simulink model "robotTask"  (R2012b)
settings: Solver=FixedStepDiscrete  StartTime=0.0  StopTime=10.0  FixedStep=0.001  RelTol=1e-3
undefined symbols (not defined in the file): acquireMethods, autoplayMovementDuration, autoplayReactionTime, autoplayRotationDuration, autoplayRotationStart, centerOffset, clickPercentage, clickRefractoryPeriod, clickTargetColor, clickTargetHoverColor, cuedText, cuedTextLength, cumulativeDwell, cursorColorClick, cursorColorClosed, cursorColorOpen, cursorDiameter, cursorNeuralColor, cursorNonneuralColor, delayOrder, delayPeriodGainScale, displayObject, doHeadSpeedFail, drawNumbersOnTargets, dwellRefractoryPeriod, errorAssistAxis, errorAssistR, errorAssistTheta, expRandBinSize, expRandMax, expRandMin, expRandMu, eyeMode, failOnLiftoff, failurePenalty, falseClickFails, fingerPositionTolerance, fixedSeqMode, freePlayMode, gain, gloveBias, gloveLPDenominator, gloveLPNumerator, gloveNonlinearCorrection, gloveXCorrection, gloveYCorrection, gridEdges, gridTilesEachDim, headSpeedCap, holdDuration, holdTime, initialInput, initialLockout, initialState, inputType, keyboard, keyboardDims, keyPressedTime, lockFingerPosition, maxTaskTime ... (+100)
(part 2 of 2)

== matlab function robotTask/robotTaskSplit ==
  data: xkRaw input double size=[double(xkConstants.NUM_STATE_DIMENSIONS) 1]; xkMod input; behaviorPacket input Bus: behaviorPacketBus size=1; vizData input Bus: peripheralData; clickState input; clickParameters input; taskOutput output Bus: taskOutput; stateParameters input Bus: stateParams size=1; taskParameters input Bus: taskParamsBus; clock input; xpcTET input; xkModBiasEst input; taskAgnosticXk input
function taskOutput  = robotTaskSplit(xkRaw, xkMod, behaviorPacket, vizData, clickState, clickParameters, stateParameters, taskParameters, clock, xpcTET, xkModBiasEst, taskAgnosticXk)
%#codegen
% This is the state-machine-like implementation of the robot task. 
% It was originally cloned from cursorTask, but my goal is to strip out the
% unused task logic in preparation for having future robotic tasks.
% 
% This also does some robot-specific things like using the click selection
% to implement grasp logic. 
%
% It two state inputs, xkRaw (which gets fed back to
% the decoder), and xkMod. Generally should look at xkMod for task logic,
% but if the game needs to change a state element which ought to propogate
% into the decoder (for example re-seed the cursor), it should do this to
% both xkRaw and xkMod.

% taskParameters is taskParamsBus, which is set by
% robotTask_buildWorkspace.m

robotPosition = behaviorPacket.robotPosition; % 1x3 of x y z % SDS I *think* but need to check that this is the returned position of robot
behaviorRequestClock = behaviorPacket.xpcRequestClock;
peripheralTimestamp = behaviorPacket.peripheralTimestamp(1:16);

%% CONSTANTS
TASK_NAME = 'robot';
VERSION_ID = single(1); % v1 is Feb 2017
NUM_DIMS = uint8(cursorConstants.NUM_DIMENSIONS); % dimensionality of the task. August 2016 raised this from 2 to 3
STATEVEC_SIZE = double( xkConstants.NUM_STATE_DIMENSIONS ); % SDS July 2016
INIT_LENGTH = uint16(100); %ms
PRE_TRIAL_LENGTH = uint16(20); %ms
INIT_TIME = uint32(2000);


%% INITIALIZE CURSOR TASK OUTPUT
fileLoggerData.data = uint8(zeros(1,1400));
fileLoggerData.dataLen = uint16(0);
fileLoggerData.fileName = uint8(zeros(1,20));
fileLoggerData.send = false;

fileLoggerFormat.format = uint8(zeros(1,1400));
fileLoggerFormat.formatLen = uint16(0);
fileLoggerFormat.fileName = uint8(zeros(1,20));

fileLoggerFormatAndData.format = fileLoggerFormat;
fileLoggerFormatAndData.data = fileLoggerData;

%% whether or not to allow the cursor to be stopped (e.g. during click)
allowStop = true;
resetHMM = false;

taskOutput.flushFiles = false;
taskOutput.sendFormat = false;
taskOutput.taskDetails = fileLoggerFormat;
taskOutput.discrete = fileLoggerFormatAndData;
taskOutput.continuous = fileLoggerFormatAndData;
taskOutput.screen = fileLoggerFormatAndData;
taskOutput.sound = fileLoggerFormatAndData;
taskOutput.asynch = fileLoggerFormatAndData;
taskOutput.ttl = double(0);
taskOutput.xk = xkRaw;
taskOutput.inputType = taskParameters.initialInput;
% initial target is off-screen
taskOutput.currentTarget = single(999.*ones([double(xkConstants.NUM_TARGET_DIMENSIONS) 1]));
taskOutput.state = uint16(CursorStates.STATE_INIT);
taskOutput.paused = false;
taskOutput.allowStop = allowStop;
taskOutput.resetHMM = resetHMM;

%% TASK DETAILS PACKET
taskOutput.taskDetails = packFileLoggerTaskDetails(TASK_NAME, VERSION_ID, ...
    'STATE_INIT', uint8(CursorStates.STATE_INIT), ...
    'STATE_PRE_TRIAL', uint8(CursorStates.STATE_PRE_TRIAL),...
    'STATE_NEW_TARGET', uint8(CursorStates.STATE_NEW_TARGET),...
    'STATE_MOVE', uint8(CursorStates.STATE_MOVE),...
    'STATE_ACQUIRE', uint8(CursorStates.STATE_ACQUIRE),...
    'STATE_SUCCESS', uint8(CursorStates.STATE_SUCCESS),...
    'STATE_FAIL', uint8(CursorStates.STATE_FAIL),...
    'STATE_CENTER_TARGET', uint8(CursorStates.STATE_CENTER_TARGET),...
    'STATE_END', uint8(CursorStates.STATE_END),...
    'STATE_RECENTER_DELAY', uint8(CursorStates.STATE_RECENTER_DELAY),...
    'STATE_MOVE_CLICK', uint8(CursorStates.STATE_MOVE_CLICK),...
    'STATE_MOVE_HOVER', uint8(CursorStates.STATE_HOVER),...
    'CLICK_IDLE', uint8(DiscreteStates.CLICK_IDLE),...
    'CLICK_MAIN', uint8(DiscreteStates.CLICK_MAIN),...
    'TARGET_TYPE_DWELL', uint8(cursorConstants.TARGET_TYPE_DWELL), ...
    'TARGET_TYPE_CLICK', uint8(cursorConstants.TARGET_TYPE_CLICK), ...
    'INPUT_TYPE_MOUSE_ABSOLUTE', uint8(cursorConstants.INPUT_TYPE_MOUSE_ABSOLUTE),...
    'INPUT_TYPE_DECODE_V', uint8(cursorConstants.INPUT_TYPE_DECODE_V),...
    'INPUT_TYPE_AUTO_PLAY', uint8(cursorConstants.INPUT_TYPE_AUTO_PLAY),...
    'CLICK_TYPE_NONE', uint8(clickConstants.CLICK_TYPE_NONE),...
    'CLICK_TYPE_NEURAL', uint8(clickConstants.CLICK_TYPE_NEURAL),...
    'OUTPUT_TYPE_CURSOR', uint8(cursorConstants.OUTPUT_TYPE_CURSOR),...
    'OUTPUT_TYPE_ROBOT', uint8(cursorConstants.OUTPUT_TYPE_ROBOT)...
);



%% DEFINE PERSISTENTS
persistent state vizPacket;
persistent pauseTriggered;
persistent stateTimer;
persistent holdTimer;
persistent clickTimer; %added SDS Jan 2017, so both click and hold can be used to do this task
persistent cursorColors;

persistent currentTarget;
persistent nextTarget;

persistent currentTargetType nextTargetType;  % dwell or click
persistent trialNum targetOrder cycleNum cycleIndex;
persistent trialDelayLength;

persistent localAcquired localTotal localTotalTime localAcqTime;
persistent acquireTime lastState;

persistent lockedParameters inputType outputType;
persistent stateBeforePreTrial;

persistent lastSoundTime;
persistent lastSoundState;

persistent initialCursorPosition previousInput;

persistent totalTaskTime;
persistent lastAcquireSuccess previousTarget;

%% INITIALIZE PERSISTENTS
if(isempty(state))
    state = uint16(CursorStates.STATE_INIT);
    lastState = state;
    % initial current target is off screen
    currentTarget = single(999.*ones([double(xkConstants.NUM_TARGET_DIMENSIONS) 1]));
    nextTarget = single(zeros([double(xkConstants.NUM_TARGET_DIMENSIONS) 1]));

    
    vizPacket = initVizPacket;
    stateTimer = uint16(0);
    holdTimer = int16(0);
    clickTimer = int16(0); % initialize
    pauseTriggered = true;
    
    cursorColors = double(zeros([3 2])); % there's a second cursor (column 2) allowed
    
    
    %% buffer all the parameters off the bus
    lockedParameters = taskParameters;
    
    
    inputType = lockedParameters.initialInput;
    
    targetOrder = uint16(zeros([1 double(cursorConstants.MAX_TARGETS)]));
    trialNum = uint16(0);
    cycleNum = uint16(0);
    cycleIndex = uint16(0);
    trialDelayLength = uint16(0);
    
    localTotal = uint16(0);
    localTotalTime = uint16(0);
    localAcquired = uint16(0);
    localAcqTime = uint16(0);
    localScore = uint16(0);
    totalScore = uint16(0);
    acquireTime = stateTimer;
    currentTargetType = uint16(cursorConstants.TARGET_TYPE_DWELL);
    nextTargetType = uint16(cursorConstants.TARGET_TYPE_DWELL);
	stateBeforePreTrial = uint16(0);
    lastSoundTime = clock;
    lastSoundState = uint8(CursorStates.SOUND_STATE_IDLE);
    
    initialCursorPosition = zeros(NUM_DIMS,1);
    previousInput = inputType;
    
    totalTaskTime = uint32(0);
    
    lastAcquireSuccess = false;
    previousTarget = currentTarget;
end


%% some initialization
if(clock < INIT_TIME)
    pauseTriggered = true;
end
outputType = lockedParameters.outputType; % determines what graphics engine will render this task.

% We usually shouldn't write discrete data
writeDiscreteData = false;
writeContinuousData = true;

if(vizData.receive && (vizData.dataLen > 0 ))
    vizPacket = parseVizPacket(vizData.data);
end

isNeural = (uint16(inputType) == uint16(cursorConstants.INPUT_TYPE_DECODE_V));
isClicked = (uint16(clickState) == uint16(DiscreteStates.CLICK_MAIN));
if ~isClicked
    clickTimer = int16(0); % resets t be not-clicked
end
isNone = (uint16(inputType) == uint16(cursorConstants.INPUT_TYPE_NONE));

% which state elements do I look to for the cursor's position? SDS July 2016
xk2HorizontalPos = uint8( lockedParameters.xk2HorizontalPos );
xk2VerticalPos = uint8( lockedParameters.xk2VerticalPos );
xk2HorizontalVel = uint8( lockedParameters.xk2HorizontalVel );
xk2VerticalVel = uint8( lockedParameters.xk2VerticalVel );
xk2DepthPos = uint8( lockedParameters.xk2DepthPos );
xk2DepthVel = uint8( lockedParameters.xk2DepthVel );
xk2RotatePos = uint8( lockedParameters.xk2RotatePos );
xk2RotateVel = uint8( lockedParameters.xk2RotateVel );
xk2Rotate2Pos = uint8( lockedParameters.xk2Rotate2Pos );
xk2Rotate2Vel = uint8( lockedParameters.xk2Rotate2Vel );

canBePosInds = [xk2HorizontalPos,xk2VerticalPos,xk2DepthPos,xk2RotatePos,xk2Rotate2Pos];
canBeVelInds = [xk2HorizontalVel,xk2VerticalVel,xk2DepthVel,xk2RotateVel,xk2Rotate2Vel];
effectorPosInds = canBePosInds(1:NUM_DIMS);
effectorVelInds = canBeVelInds(1:NUM_DIMS);

if uint16(outputType) == uint16(cursorConstants.OUTPUT_TYPE_ROBOT)
    effectorPos = double(robotPosition(1:2)); % MAKE N-D
    % TODO: when we start doing simulated/real arms, work on this stuff
elseif uint16(outputType) == uint16(cursorConstants.OUTPUT_TYPE_SCLCURSOR)
    effectorPos = xkMod(effectorPosInds);
else
    effectorPos = xkMod(effectorPosInds);
end


%% set the cursor color 
if isClicked
    cursorColors(1:end,1) = lockedParameters.cursorColorClick;%[255; 0; 0;];
elseif isNeural
    cursorColors(1:end,1) = [255; 255; 255;]; % white neural cursor
elseif isNone
    cursorColors(1:end,1) = [0; 204; 102;]; % is this used?
else
    cursorColors(1:end,1) = [255; 133; 0]; % orange autoplay cursor
end


targetColor = 'g';



if ~pauseTriggered
    totalTaskTime = totalTaskTime+1;
end

%% generally, allow cursor to stop off target. check options
allowStop = lockedParameters.stopOffTarget;

% STATE MACHINE
switch state
    %% STATE_INIT
    case {CursorStates.STATE_INIT}
        % set all the persistents that may have been changed by user input
        pauseTriggered = stateParameters.pause;
        lockedParameters = taskParameters;
        writeContinuousData = false;
        inputType = lockedParameters.initialInput;
        % generate some entropy
        jnk = rand(1,1);
        
        initialCursorPosition = xkMod(effectorPosInds(1:NUM_DIMS)); % handhold the compiler so it knows its fixed dim.
        if ~pauseTriggered
            stateTimer = stateTimer + 1;
        end
        if stateTimer >= INIT_LENGTH
            stateTimer = uint16(0);
            trialNum = uint16(0);
            % Initialize without a target, so jjust put it somewhere far
            % away            
            currentTarget(:) = int16(999.*ones(double(xkConstants.NUM_TARGET_DIMENSIONS),1));
            cycleNum = uint16(0);
            
            % For robot task, go straight to STATE_MOVE or
            % STATE_MOVE_CLICK
            %
            state = uint16( RobotStates.STATE_PRE_TRIAL );
            % Key logic for whether to go into STATE_MOVE or
            % STATE_MOVE_CLICK, based on what mode is selected,
%             if currentTargetType == cursorConstants.TARGET_TYPE_CLICK;
%                 state = uint16(RobotStates.STATE_MOVE_GRASP_OPEN);
%             elseif currentTargetType == cursorConstants.TARGET_TYPE_DWELL;
%                 state = uint16(RobotStates.STATE_MOVE);
%             end
        end
        
        
        %% STATE_CENTER_TARGET
    case {RobotStates.STATE_CENTER_TARGET}
        stateTimer = stateTimer + 1;
        initialCursorPosition = xkMod(effectorPosInds(1:NUM_DIMS)); % the (1:NUM_DIMS) is to handhold compilter about the dimensionality  
        if isCursorOnTarget(effectorPos, double(lockedParameters.cursorDiameter)/2, currentTarget, double(lockedParameters.targetDiameter)/2, NUM_DIMS)
            state = uint16(RobotStates.STATE_SUCCESS);
            stateTimer = uint16(0);
        end
        
        
        
        %% STATE_NEW_TARGET
    case {RobotStates.STATE_NEW_TARGET}
        holdTimer = int16(0); % reset hold timer. Needed now for Gridlike task logic SDS 15 Dec 2016
        
        if ~trialDelayLength
            if lockedParameters.useRandomDelay
                % pick a new random delay
                while double(trialDelayLength) < lockedParameters.expRandMin || double(trialDelayLength) > lockedParameters.expRandMax
                    trialDelayLength = uint16(lockedParameters.expRandMu * -log(rand([1 1])));
                end
                trialDelayLength = uint16(round(double(trialDelayLength) / double(lockedParameters.expRandBinSize))*lockedParameters.expRandBinSize);
            else
                trialDelayLength = uint16(lockedParameters.expRandMu);
            end
        end
        
        % Check whether cursor is in target differs for Gridlike task.
        cursorOnTarget = isCursorOnTarget(effectorPos, double(lockedParameters.cursorDiameter)/2,  currentTarget, double(lockedParameters.targetDiameter)/2, NUM_DIMS);
        
        stateTimer = stateTimer + 1;
        if stateTimer >= trialDelayLength
            % great, present the new target now
            stateTimer = uint16(0);
            previousTarget = currentTarget;
            currentTarget = nextTarget;
            currentTargetType = nextTargetType;

            % is recentering turned on, and does that apply here?
            if (lockedParameters.recenterOnSuccess && lastAcquireSuccess ==true ) || ...
                    (lockedParameters.recenterOnFail && lastAcquireSuccess == false)
                recenterThisTrial = true;
            else
                recenterThisTrial = false;
            end
            
            if recenterThisTrial
                state = uint16(RobotStates.STATE_RECENTER_DELAY);
            else
                if lockedParameters.soundOnGo
                    lastSoundTime = clock;
                    lastSoundState = uint8(RobotStates.SOUND_STATE_GO);
                end
                % Key logic for whether to go into STATE_MOVE or
                % one of the move-and-grasp states
                if currentTargetType == cursorConstants.TARGET_TYPE_CLICK;
                    state = uint16(RobotStates.STATE_MOVE_GRASP_OPEN);
                elseif currentTargetType == cursorConstants.TARGET_TYPE_DWELL;
                    state = uint16(RobotStates.STATE_MOVE);
                end
            end
        elseif ~cursorOnTarget 
            % Note that there's no stay-over-target rule for Gridlike
            % task, so in that task this won't be reached.
            % For other task variants: if cursor moves from last target too early,
            % just reset delay timer
            stateTimer = uint16(0);
        end
        
        %% STATE_RECENTER_DELAY
    case {RobotStates.STATE_RECENTER_DELAY}
        % (Gridlike task variant never enters this state)
        % Not currently used in robot task either.
        stateTimer = stateTimer + 1;
        if stateTimer <= lockedParameters.recenterDelay
            switch lockedParameters.taskType
                case {uint32(cursorConstants.TASK_PINBALL), ...
                        uint32(cursorConstants.TASK_CENTER_OUT)}                       
                    xkMod(effectorPosInds,1) = previousTarget(1:NUM_DIMS);
                    xkMod(effectorVelInds,1) = 0;
                case uint32(cursorConstants.TASK_CENTER_OUT_NO_BACK)
                    xkMod([effectorPosInds, effectorVelInds],1) = 0;
                case uint32(cursorConstants.TASK_NOTARGETS)
                    % go back to workspace center
                    xkMod([effectorPosInds, effectorVelInds],1) = 0;
            end
            xkRaw([effectorPosInds, effectorVelInds],1) = xkMod([effectorPosInds, effectorVelInds],1); % also lock xkRaw
        else
            if lockedParameters.soundOnGo
                lastSoundTime = clock;
                lastSoundState = uint8(RobotStates.SOUND_STATE_GO);
            end
            
            stateTimer = uint16(0);
            if currentTargetType == cursorConstants.TARGET_TYPE_CLICK;
                state = uint16(RobotStates.STATE_MOVE_GRASP_OPEN);
            elseif currentTargetType == cursorConstants.TARGET_TYPE_DWELL;
                state = uint16(RobotStates.STATE_MOVE);
            end
        end
        
        %% STATE_MOVE
    case {RobotStates.STATE_MOVE}
        % moving and no grasp control
        stateTimer = stateTimer + 1;
        inputType = lockedParameters.inputType; % needed to unlock cursor if not coming from success state
        

        cursorOnTarget = isCursorOnTarget(effectorPos, double(lockedParameters.cursorDiameter)/2,  currentTarget, double(lockedParameters.targetDiameter)/2, NUM_DIMS);

        if cursorOnTarget
            state = uint16(RobotStates.STATE_ACQUIRE);
            if holdTimer >= 0
                holdTimer = int16(0); % reset hold timer -- it could have been nonzero from either previous
                % target hold or time spent in any tile in Gridlike mode.
            else
                holdTimer = holdTimer; % allows negative to carry over for newTrialAddedDwell
            end
            
            if lockedParameters.soundOnOverTarget
                % if we're on autoplay, make a tapping noise
                lastSoundTime = clock;
                lastSoundState = uint8(RobotStates.SOUND_STATE_OVER_TARGET);
            end
        elseif stateTimer >= lockedParameters.trialTimeout
            stateTimer = uint16(0);
            state = uint16(RobotStates.STATE_FAIL);
        end

        
        
    %% STATE_MOVE_GRASP_OPEN
    case {RobotStates.STATE_MOVE_GRASP_OPEN}
        stateTimer = stateTimer + 1;
        inputType = lockedParameters.inputType; % needed to unlock if not coming from success
        
        
        networkOutput.discrete.send = false; % SDS: not really sure why this is set here but not in e.g. STATE_MOVE
        
        cursorOnTarget = isCursorOnTarget(effectorPos, double(lockedParameters.cursorDiameter)/2,  currentTarget, double(lockedParameters.targetDiameter)/2, NUM_DIMS);
        targetColor = 'y';
        % Shows hand should be open based on cursor color (useful for SCL
        % testing).
        cursorColors(1:end,1) = lockedParameters.cursorColorOpen;
        
        if clickState == uint16(DiscreteStates.CLICK_MAIN)
            clickTimer = clickTimer + 1;
            if clickTimer >= clickParameters.clickHoldTime && stateTimer > taskParameters.selectionRefractoryMS
                % Click command was sent into the task long enough that the
                % toggle is triggered, AND we've been in this state longer
                % than the refractory period (this debounces state
                % transitions).
                state = uint16( RobotStates.STATE_MOVE_GRASP_CLOSED );
                stateTimer = uint16(0);
            end
        end
        
        
        if cursorOnTarget
            state = uint16(RobotStates.STATE_HOVER);
            if holdTimer >= 0
                holdTimer = int16(0); % reset hold timer -- it could have been nonzero from either previous
                % target hold or time spent in any tile in Gridlike mode.
            else
                holdTimer = holdTimer; % allows negative to carry over for newTrialAddedDwell
            end
            
            if lockedParameters.soundOnOverTarget
                % if we're on autoplay, make a tapping noise
                lastSoundTime = clock;
                lastSoundState = uint8(RobotStates.SOUND_STATE_OVER_TARGET);
            end
            
        elseif stateTimer >= lockedParameters.trialTimeout
            stateTimer = uint16(0);
            state = uint16(RobotStates.STATE_FAIL);
        end
        
  %% STATE_MOVE_GRASP_CLOSED
    case {RobotStates.STATE_MOVE_GRASP_CLOSED}
        stateTimer = stateTimer + 1;
        inputType = lockedParameters.inputType; % needed to unlock if not coming from success
        
        
        networkOutput.discrete.send = false; % SDS: not really sure why this is set here but not in e.g. STATE_MOVE
        
        cursorOnTarget = isCursorOnTarget(effectorPos, double(lockedParameters.cursorDiameter)/2,  currentTarget, double(lockedParameters.targetDiameter)/2, NUM_DIMS);
        targetColor = 'y';
        % Shows hand should be open based on cursor color (useful for SCL
        % testing).
        cursorColors(1:end,1) = lockedParameters.cursorColorClosed;
        
         if clickState == uint16(DiscreteStates.CLICK_MAIN)
            clickTimer = clickTimer + 1;
            if clickTimer >= clickParameters.clickHoldTime && stateTimer > taskParameters.selectionRefractoryMS
                % Click command was sent into the task long enough that the
                % toggle is triggered, AND we've been in this state longer
                % than the refractory period (this debounces state
                % transitions).
                state = uint16( RobotStates.STATE_MOVE_GRASP_OPEN );
                stateTimer = uint16(0);
            end
        end
        
        if cursorOnTarget
            state = uint16(RobotStates.STATE_HOVER);
            if holdTimer >= 0
                holdTimer = int16(0); % reset hold timer -- it could have been nonzero from either previous
                % target hold or time spent in any tile in Gridlike mode.
            else
                holdTimer = holdTimer; % allows negative to carry over for newTrialAddedDwell
            end
            
            if lockedParameters.soundOnOverTarget
                % if we're on autoplay, make a tapping noise
                lastSoundTime = clock;
                lastSoundState = uint8(RobotStates.SOUND_STATE_OVER_TARGET);
            end
            
        elseif stateTimer >= lockedParameters.trialTimeout
            stateTimer = uint16(0);
            state = uint16(RobotStates.STATE_FAIL);
        end       
        
        %% STATE_HOVER
    case {RobotStates.STATE_HOVER}
        % Hover is being over a target when click enabled - Sergey
        stateTimer = stateTimer + 1;
        % SDS Jan 26 2017. I'm making hold to select possible in cursor
        % task, even when click is also an option. Hence, now holdTimer
        % counts up here too.
        holdTimer = holdTimer + 1;
        
        % if "stopOffTarget" is false, then we must manually
        %   flag times when cursor is over target to allow click to stop
        allowStop = true;
        
        networkOutput.discrete.send = false;
        
        cursorOnTarget = isCursorOnTarget(effectorPos, double(lockedParameters.cursorDiameter)/2,  currentTarget, double(lockedParameters.targetDiameter)/2, NUM_DIMS);
        targetColor = 'p';
        
        if clickState == uint16(DiscreteStates.CLICK_MAIN)
            clickTimer = clickTimer + 1;
            if clickTimer >= clickParameters.clickHoldTime % should be clickTimer
                if holdTimer > 0
                    % above check is the refractory period.
                    if cursorOnTarget
                        state = uint16(RobotStates.STATE_SUCCESS);
                        stateTimer = uint16(0);
                    else
                        state = uint16(RobotStates.STATE_FAIL);
                        stateTimer = uint16(0);
                        %  holdTimer = int16(0);  % should be clickTimer
                    end
                end
            end
            
        elseif ~cursorOnTarget
            % the elseif means that if mid-click and drifting off a
            % target, that's not yet a fail. But if NOT still clicking,
            % and drift off a target, then it goes to STATE_MOVE_CLICK.
            % Note that due to logic above in the click check, gridlike
            % task is less forgiving.
            state = uint16(RobotStates.STATE_MOVE_GRASP_OPEN);
            % TODO: need to think about what state to move to after an
            % incorrect grasp command. Maybe irrelevant if we don't end up
            % using this
            
            % we were over the target, but now we're not, so either
            % left target (vanilla cursor task) or the tile (gridlike).
            % Either way, hold timer becomes zero if nonnegative/
            if holdTimer > 0
                % this check > 0 is so that rapidly fluttering over
                % target in gridlike task doesn't nullify refractory
                % period.
                holdTimer = int16(0);
            end
        elseif holdTimer >= lockedParameters.holdTime
            % held over the target long enough to acquire it
            acquireTime = stateTimer;
            stateTimer = uint16(0);
            state = uint16(RobotStates.STATE_SUCCESS);
            holdTimer = int16(0);
            
        elseif stateTimer >= lockedParameters.trialTimeout
            stateTimer = uint16(0);
            state = uint16(RobotStates.STATE_FAIL);
            holdTimer = int16(0);  % should be clickTimer
            
        else
            clickTimer = int16(0);    % should be clickTimer
            % likely redundant to check at top of the function, but
            % can't hurt here.
        end
        
        %% STATE_ACQUIRE
    case {RobotStates.STATE_ACQUIRE}
        stateTimer = stateTimer + 1;
        holdTimer = holdTimer + 1;
        % if "stopOffTarget" is false, then we must manually
        %   flag times when cursor is over target to allow click to stop
        
        % Check whether cursor is in target differs for Gridlike task.
        cursorOnTarget = isCursorOnTarget(effectorPos, double(lockedParameters.cursorDiameter)/2,  currentTarget, double(lockedParameters.targetDiameter)/2, NUM_DIMS);
        targetColor = 'b';

        allowStop = true;
        
        if ~cursorOnTarget
            state = uint16(RobotStates.STATE_MOVE);
            if holdTimer > 0
                % check for > 0 so briefly entering and exiting a
                % target doesn't void negative holdTime that is used as
                % a refractory period.
                holdTimer = int16(0);
            end
        elseif holdTimer >= lockedParameters.holdTime
            acquireTime = stateTimer;
            stateTimer = uint16(0);
            state = uint16(RobotStates.STATE_SUCCESS);
        end
        
        %% STATE_SUCCESS
    case {RobotStates.STATE_SUCCESS}
        inputType = lockedParameters.inputType;
        trialNum = trialNum+1;
        
        % how do we score this trial?
        localTotal = localTotal+1;
        localAcquired = localAcquired + 1;
        localTotalTime = localTotalTime + acquireTime;
        
        localAcqTime = uint16(single(localTotalTime) / single(localTotal));
        lastAcquireSuccess = true;
        
        stateTimer = uint16(0);
        if lockedParameters.soundOnSuccess
            lastSoundTime = clock;
            lastSoundState = uint8(RobotStates.SOUND_STATE_SUCCESS);
        end
       
        state = uint16(RobotStates.STATE_PRE_TRIAL);
        
        % if we've finished a cycle, start a new cycle ("chain" in rigC
        % parlance).
        % SDS Dec 2016, trying to make sense of this.
        % cycleIndex tracks which cycle we're on. So e.g. if there's an
        % 8 target cycle, we might do ~5 cycles in a block (40 trials).
        % targetInds has the coordiantes of targets, it is set in the
        % parameter scripts. numTargets is e.g. 8 (for 8 Target Task),
        % and is also set in the parameter script.
        switch lockedParameters.taskType
            case {uint32(cursorConstants.TASK_PINBALL)}
                if ~mod(trialNum-1, lockedParameters.numTargets)
                    cycleNum = cycleNum+1;
                    % randomize the order of targets for the next
                    % cycle.
                    targetOrder(1:lockedParameters.numTargets) = randperm(lockedParameters.numTargets);
                end
                cycleIndex = mod(trialNum-1, lockedParameters.numTargets)+1;
                
            case {uint32(cursorConstants.TASK_CENTER_OUT_NO_BACK)}
                if ~mod(trialNum-1, lockedParameters.numTargets)
                    cycleNum = cycleNum+1;
                    % randomize the order of targets for the next
                    % cycle.
                    targetOrder(1:lockedParameters.numTargets) = randperm(lockedParameters.numTargets);
                end
                cycleIndex = mod(trialNum-1, lockedParameters.numTargets)+1;
            case {uint32(cursorConstants.TASK_CENTER_OUT)}
                if ~mod(trialNum-1, lockedParameters.numTargets*2)
                    cycleNum = cycleNum+1;
                    % Randomize the order of targets for the next
                    % cycle.
                    targetOrder(1:lockedParameters.numTargets) = randperm(lockedParameters.numTargets);
                end
                cycleIndex = uint16(floor(mod(double((trialNum-1)/2), lockedParameters.numTargets)))+1;
        end
        
        %% STATE_FAIL
    case {RobotStates.STATE_FAIL}
        stateTimer = stateTimer+1;
        lastAcquireSuccess = false;
        
        % Check whether cursor is in target differs for Gridlike task.
        cursorOnTarget = isCursorOnTarget(effectorPos, double(lockedParameters.cursorDiameter)/2,  currentTarget, double(lockedParameters.targetDiameter)/2, NUM_DIMS);
        if cursorOnTarget
            holdTimer = holdTimer + 1;
        else
            holdTimer = int16(0);
        end
        if holdTimer >= lockedParameters.failurePenalty
            trialNum = trialNum + 1;
            stateTimer = uint16(0);
            
            %% how do we score this trial?
            localTotal = localTotal+1;
            localAcqTime = uint16(single(localTotalTime) / single(localTotal));
            
            
            state = uint16(RobotStates.STATE_PRE_TRIAL);
        end
        if lockedParameters.soundOnFail
            lastSoundTime = clock;
            lastSoundState = uint8(RobotStates.SOUND_STATE_FAIL);
        end
        
        
        
        %% STATE_PRE_TRIAL
    case {RobotStates.STATE_PRE_TRIAL}
        %% capture pauses
        if stateTimer == 0
            pauseTriggered = stateParameters.pause;
            stateBeforePreTrial = lastState;
        end
        if ~pauseTriggered
            stateTimer = stateTimer + 1;
        end
        
        
        % don't do this on 0, because if we're paused, 0 will occur many many times
        if stateTimer == 1
            %% choose the next target. Here's where it comes in from task parameters bus
            lockedParameters = taskParameters;
            switch lockedParameters.taskType
                % DIFFERENT TARGET CHOOSING RULES DEPENDING ON THE TASK
                % TYPE.
                case uint32(cursorConstants.TASK_CENTER_OUT)
                    % the center target is "special" and is set here.
                    % The other targets come from
                    % lockedParameters.targetInds.
                    if mod(trialNum, 2) == 0
                        % CENTER TARGET
                        nextTarget = single(zeros( double( xkConstants.NUM_TARGET_DIMENSIONS ), 1) );
                    else
                        % OTHER TARGETS
                        nextTarget = lockedParameters.targetInds(:,targetOrder(cycleIndex));
                    end
                case uint32( cursorConstants.TASK_NOTARGETS )
%                      nextTarget = single(nan( double(
%                      xkConstants.NUM_TARGET_DIMENSIONS ), 1) ); % seems
%                      to lead to weird behavior

                    % Target is off-screen at 999
                    nextTarget = single(999.*ones( double( xkConstants.NUM_TARGET_DIMENSIONS ), 1) );

                case  uint32(cursorConstants.TASK_CENTER_OUT_NO_BACK)
                    nextTarget = lockedParameters.targetInds(:,targetOrder(cycleIndex));
                    %% reset cursor to center
                    xkMod([effectorPosInds,effectorVelInds],1) = 0;
                    % also do this to xkRaw
                    xkRaw([effectorPosInds,effectorVelInds],1) = 0;
                case  uint32(cursorConstants.TASK_PINBALL)
                    nextTarget = lockedParameters.targetInds(:,targetOrder(cycleIndex));
            end
            clickRand = rand(1,1);
            if clickRand < lockedParameters.clickPercentage
                nextTargetType = uint16(cursorConstants.TARGET_TYPE_CLICK);
            else
                nextTargetType = uint16(cursorConstants.TARGET_TYPE_DWELL);
            end
            writeDiscreteData = true;
            
        end
        if stateTimer >= PRE_TRIAL_LENGTH
            if trialNum > lockedParameters.numTrials
                %% are we done?
                state = uint16(RobotStates.STATE_END);
            else
                state = uint16(RobotStates.STATE_NEW_TARGET);
            end
            stateTimer = uint16(0);
            trialDelayLength = uint16(0);
            
        end
        
        %% STATE_END
    case {RobotStates.STATE_END}
        stateTimer = stateTimer + 1;
        % Hide the target so it's clear to participant that the task is
        % complete.
        % Added SDS Jan 2017
        currentTarget(1:end) = 9999;
        
end

if lockedParameters.maxTaskTime && totalTaskTime > lockedParameters.maxTaskTime
    state = uint16(RobotStates.STATE_END);
end


%% Special cursor position reset for robotTask
% since robot control is done through velocities, we don't use xPC
% workspace boundaries, meaning the cursor can go off-screen. In order to
% keep it somewhere visible (so operator can watch SCL cursor to see
% commanded velocities), when it goes off-screen it gets teleported back to
% center. Note this will be logged in xk so analyses will have to remember
% not to trust this.
if any( abs( xkMod(effectorPosInds) ) > 0.13 )
    xkMod(effectorPosInds,1) = 0;
    xkRaw(effectorPosInds,1) = 0;
end



taskOutput.xk = xkRaw; % feed *raw* xk back out, which goes to decoder and file logger
taskOutput.currentTarget = single(currentTarget(:,1));
taskOutput.state = state;





 

%%
cursorPosition = single(xkMod(effectorPosInds)');
cursorVelocity = single(xkMod(effectorVelInds)');
taskAgnosticVel = single(taskAgnosticXk(effectorVelInds)');

%% PACK DATA FOR UDP OUTPUT (filelogger continuous)
taskOutput.continuous = packFileLoggerFormatAndData('continuous', ...
    TASK_NAME, VERSION_ID, ...
    'clock', clock, ...
    'pause', pauseTriggered, ...
    'xpcRequestClock', behaviorRequestClock, ...
    'peripheralTimestamp', peripheralTimestamp, ...
    'state', state, ...
    'inputType', inputType, ...
    'xpcScreenUpdateClock',vizPacket.xpcScreenUpdateClock,...
    'cursorPosition', cursorPosition(1:NUM_DIMS), ...
    'taskAgnosticVel', taskAgnosticVel(1:NUM_DIMS), ...
    'currentTarget', single(currentTarget(:,1)), ...
    'currentTargetType', uint16(currentTargetType),...
    'clickState', uint16(clickState),...
    'xk', single(taskOutput.xk),...
    'stateTimer', stateTimer, ...
    'holdTimer', holdTimer, ...   
    'behaviorPacketSize', behaviorPacket.packetSize, ...
    'xpcTET', single(xpcTET), ...
    'robotTimestamp', behaviorPacket.robotTimestamp, ...
    'robotPosition', robotPosition, ...
    'gain', taskParameters.gain, ...  % not locked  
    'powerGain', taskParameters.powerGain, ...
    'powerGainUnityCrossing', taskParameters.powerGainUnityCrossing, ...
    'xkModBiasEst', single(xkModBiasEst) ...
    );





%% SEND DISCRETE DATA TO FILELOGGER
taskOutput.discrete = packFileLoggerFormatAndData('discrete', ...
    TASK_NAME, VERSION_ID, ...
    'clock', clock,...
    'blockNumber', stateParameters.blockNumber,...
    'state', state, ...
    'taskType', lockedParameters.taskType, ...
    'targetDiameter', lockedParameters.targetDiameter, ...
    'trialDelayLength', trialDelayLength, ...
    'currentTarget', currentTarget,...
    'holdTime', lockedParameters.holdTime, ...
    'clickPercentage', single(lockedParameters.clickPercentage), ...
    'hmmClickLikelihoodThreshold',clickParameters.hmmClickLikelihoodThreshold,...
    'clickHoldTime', clickParameters.clickHoldTime, ...
    'clickSource', clickParameters.clickSource, ...
    'trialNum', trialNum, ...
    'inputType', inputType, ...
    'workspaceX', lockedParameters.workspaceX, ...
    'workspacey', lockedParameters.workspaceY, ...
    'workspaceZ', lockedParameters.workspaceZ, ...
    'recenterOnSuccess', lockedParameters.recenterOnSuccess,...
    'recenterOnFail', lockedParameters.recenterOnFail,...
    'recenterDelay', lockedParameters.recenterDelay,...
    'errorAssistR',single(lockedParameters.errorAssistR),...    
    'errorAssistTheta',single(lockedParameters.errorAssistTheta),...
    'errorAssistAxis',single(lockedParameters.errorAssistTheta),... % added Oct 27 2016 SDS
    'hmmClickSpeedMax',single(clickParameters.hmmClickSpeedMax),...
    'outputType', outputType, ...
    'xk2EffectorPosInds', uint8(effectorPosInds(1:NUM_DIMS)), ...  % want to know how state is being mapped to game horizontal, veritacl, depth, rotate, ...
    'xk2EffectorVelInds', uint8(effectorVelInds(1:NUM_DIMS)), ...
    'selectionRefractoryMS', uint16( lockedParameters.selectionRefractoryMS ) ... % 
);

% SDS Removed Dec 2016 because we're up against the packet size and they're
% not currently used:
%     'gloveBias', lockedParameters.gloveBias, ...
%     'mouseOffset', lockedParameters.mouseOffset, ...
%    'nextTarget', currentTarget,...
%    'useRandomDelay', lockedParameters.useRandomDelay, ...
%    'currentTargetType', uint16(currentTargetType),...


% xk2HorizontalPos = uint8( lockedParameters.xk2HorizontalPos );
% xk2VerticalPos = uint8( lockedParameters.xk2VerticalPos );
% xk2HorizontalVel = uint8( lockedParameters.xk2HorizontalVel );
% xk2VerticalVel = uint8( lockedParameters.xk2VerticalVel );
% xk2DepthPos = uint8( lockedParameters.xk2DepthPos );
% xk2DepthVel = uint8( lockedParameters.xk2DepthVel );
% xk2RotatePos = uint8( lockedParameters.xk2RotatePos );
% xk2RotateVel = uint8( lockedParameters.xk2RotateVel );

% removed to save space , currently unused
%    'useGloveLPF', uint8(lockedParameters.useGloveLPF),...
%    'useMouseLPF', uint8(lockedParameters.useMouseLPF),...
%    'gloveThreshold', clickParameters.gloveThreshold, ...
%    'gloveIndices', clickParameters.gloveIndices, ...
%    'gloveYCorrection', single(lockedParameters.gloveYCorrection), ...
%    'gloveXCorrection', single(lockedParameters.gloveXCorrection), ...

%    'fingerPositionTolerance',single(taskParameters.fingerPositionTolerance),...
    
%% SEND DATA OUT TO VIZ
taskOutput.screen = packFileLoggerFormatAndData('screen', ...
    TASK_NAME, VERSION_ID, ...
    'clock', clock,...
    'totalTaskTime',totalTaskTime,...
    'blockNumber', stateParameters.blockNumber,...
    'state',state,...
    'cursorPosition',  horzcat(cursorPosition(1:NUM_DIMS)', nan(NUM_DIMS,1)),... % handhold the compiler with dims here
    'cursorColors', cursorColors,...
    'currentTarget', currentTarget,...
    'numTargets',uint8(lockedParameters.numTargets), ...
    'cursorDiameter', lockedParameters.cursorDiameter,...
    'targetDiameter', lockedParameters.targetDiameter,...
    'targetColor', targetColor, ...
    'localAcquired', localAcquired,...
    'localTotal', localTotal,...
    'localAcqTime', localAcqTime,...
    'inputType', inputType,...
    'taskType', lockedParameters.taskType,...
    'recenterDelay', lockedParameters.recenterDelay,...
    'cursorVelocity', cursorVelocity(1:NUM_DIMS), ...   
    'outputType', outputType, ...
    'numDisplayDims', lockedParameters.numDisplayDims, ...
    'displayObject', lockedParameters.displayObject ... % not logged
    );

%% SEND DATA OUT TO SOUND
taskOutput.sound = packFileLoggerFormatAndData('screen', ...
    TASK_NAME, VERSION_ID, ...
    'clock', clock,...
    'vizState',state,...
    'lastSoundTime',lastSoundTime,...
    'lastSoundState',lastSoundState...
    ); 


%% SET SEND FLAGS FOR NETWORK OUTPUTS
if(clock < INIT_TIME)
    taskOutput.discrete.data.send = false;
    taskOutput.continuous.data.send = false;
    taskOutput.screen.data.send = false;
    taskOutput.sound.data.send = false;
    
    if(mod(clock, 10)==0)
        taskOutput.sendFormat = true;
    else
        taskOutput.sendFormat = false;
    end
    stateTimer = uint16(0);
else
    taskOutput.discrete.data.send = writeDiscreteData;
    taskOutput.continuous.data.send = writeContinuousData;
    taskOutput.screen.data.send = true;
    taskOutput.sound.data.send = true;
    taskOutput.sendFormat = false;
    taskOutput.inputType = inputType;
end
taskOutput.paused = pauseTriggered;
taskOutput.allowStop = allowStop;
taskOutput.wiaCode = uint16(0);
taskOutput.speedCode = uint16(0);
lastState = state;

end



function vizPacket = parseVizPacket(packetData)

    vizPacket.xpcScreenUpdateClock = typecast(packetData(28+[1:4]), 'uint32');

end

function vizPacket = initVizPacket()

    vizPacket.xpcScreenUpdateClock = uint32(0);

end




function icot = isCursorOnTarget(effectorPos, cursorRadius, targetPosition, targetRadius, NUM_DIMS)
    % boundary checking for dims 4+ will be handled separately for the 3d
    % translational dimensions
    if NUM_DIMS > 3
        useDims = 3;
    else
        useDims = NUM_DIMS;
    end

    if sqrt( sum( ((double( effectorPos(1:useDims) ) - double( targetPosition(1:useDims) )).^2 ) ) ) < ...
            double(cursorRadius+targetRadius)
        icot = true;
    else
        icot = false;
    end
end
